simulink model "stellaris_test_pil"  (R2012b)
settings: Solver=FixedStepDiscrete  StartTime=0.0  StopTime=inf  FixedStep=0.1  RelTol=1e-3
settings Model: Creator=peselnikmg  LastModifiedBy=peselnikmg
settings DataIOCC: SignalLoggingSaveFormat=ModelDataLogs
settings OptimizationCC: OptimizeModelRefInitCode=on  LifeSpan=1
settings HardwareCC: ProdEndianess=LittleEndian  ProdHWDeviceType=Texas Instruments->TMS470
settings RTWCC: SystemTargetFile=stellaris.tlc  TemplateMakefile=stellaris_tmf  PostCodeGenCommand=stellaris_customcode(buildInfo)  Description=TI Stellaris LaunchPad  ProcessScript=stellaris_make_rtw_hook
settings CodeAppCC: IgnoreCustomStorageClasses=off
settings STFCustomTargetCC: CodeReplacementLibrary=ANSI_C  CombineOutputUpdateFcns=on  ERTCustomFileBanners=on  SupportContinuousTime=off  SupportNonInlinedSFcns=off  GRTInterface=off  SystemTargetFile=stellaris.tlc
settings ERTTargetCC: CodeReplacementLibrary=ANSI_C  MultiwordLength=2048  ParMdlRefBuildCompliant=off  CompOptLevelCompliant=off  ConcurrentExecutionCompliant=off  ERTFirstTimeCompliant=off  ModelStepFunctionPrototypeControlCompliant=off  CPPClassGenCompliant=off  InlinedParameterPlacement=NonHierarchical  ERTCustomFileTemplate=stellaris_srmain.tlc  ConvertIfToSwitch=off  SuppressUnreachableDefaultCases=off

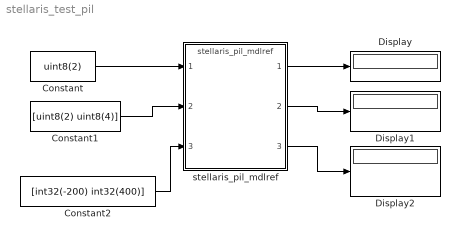
== system stellaris_test_pil ==
  Constant : Constant  Value=uint8(2)  SampleTime=0.1
  Constant1 : Constant  Value=[uint8(2) uint8(4)]  SampleTime=0.1
  Constant2 : Constant  Value=[int32(-200) int32(400)]  SampleTime=0.1
  Display : Display
  Display1 : Display
  Display2 : Display
  stellaris_pil_mdlref : ModelReference  ModelNameDialog=stellaris_pil_mdlref  SimulationMode=Processor-in-the-loop (PIL)  ModelReferenceVersion=1.11  CopyOfModelName=stellaris_pil_mdlref  DefaultDataLogging=on
  wires:
  stellaris_pil_mdlref/1 -> Display/1
  Constant/1 -> stellaris_pil_mdlref/1
  Constant1/1 -> stellaris_pil_mdlref/2
  stellaris_pil_mdlref/2 -> Display1/1
  stellaris_pil_mdlref/3 -> Display2/1
  Constant2/1 -> stellaris_pil_mdlref/3
